simulink library "SEL751_SignalScaling_lib"  (Simulink 8.1)
settings: Solver=ode45  StartTime=0.0  StopTime=10.0  RelTol=1e-3
settings Model: Creator=RE25624  LastModifiedBy=re25624

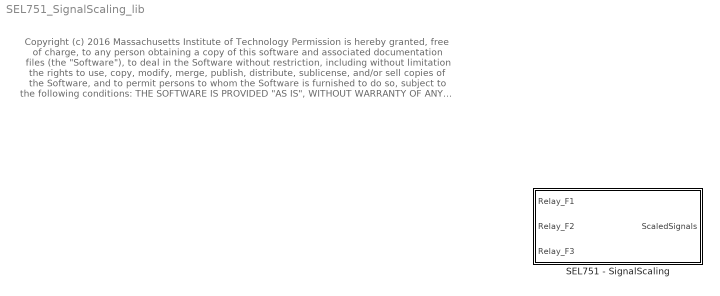
== system SEL751_SignalScaling_lib ==
  note: Copyright (c) 2016 Massachusetts Institute of Technology
      | Permission is hereby granted, free of charge, to any person obtaining a copy of this software and associated documentation files (the "Software"), to deal
      | in the Software without restriction, including without limitation the rights to use, copy, modify, merge, publish, distribute, sublicense, and/or sell copies of the
      | Software, and to permit persons to whom the Software is furnished to do so, subject to the following conditions:
      |
      | THE SOFTWARE IS PROVIDED "AS IS", WITHOUT WARRANTY OF ANY KIND, EXPRESS OR IMPLIED, INCLUDING BUT NOT LIMITED TO THE
      | WARRANTIES OF MERCHANTABILITY, FITNESS FOR A PARTICULAR PURPOSE AND NONINFRINGEMENT. IN NO EVENT SHALL THE AUTHORS
      | OR COPYRIGHT HOLDERS BE LIABLE FOR ANY CLAIM, DAMAGES OR OTHER LIABILITY, WHETHER IN AN ACTION OF CONTRACT, TORT OR
      | OTHERWISE, ARISING FROM, OUT OF OR IN CONNECTION WITH THE SOFTWARE OR THE USE OR OTHER DEALINGS IN THE SOFTWARE
  SEL751 - SignalScaling : Subsystem  mask(SEL751 - SignalScaling){ct_ratio=1/1250, pt_ratio=1/1800}
      mask prompts: ct_ratio "CT Ratio"; pt_ratio "PT Ratio"
      mask help: CT and PT ratios should match the settings in the corresponding SEL751

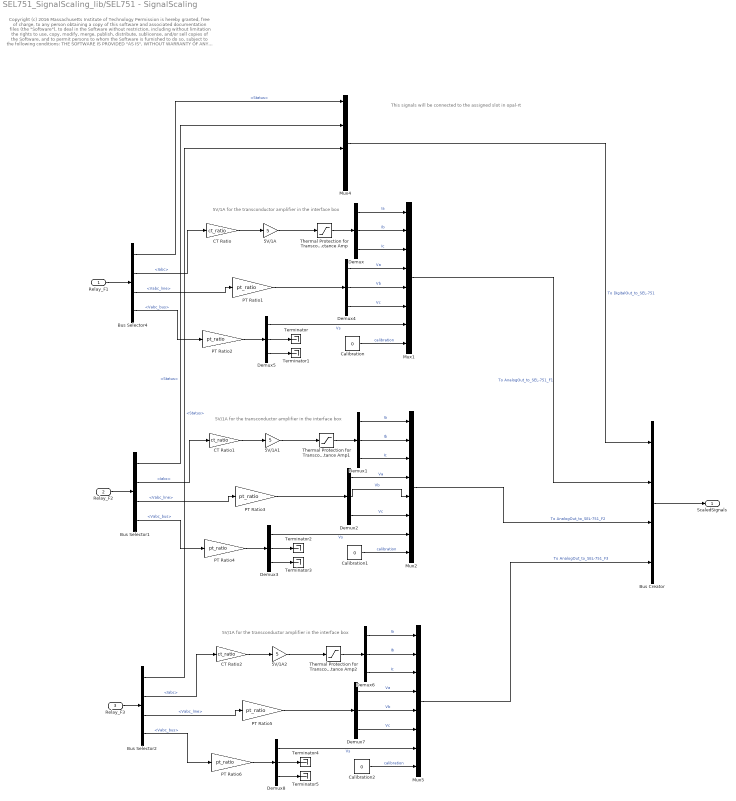
== system SEL751_SignalScaling_lib/SEL751 - SignalScaling ==
  note: Copyright (c) 2016 Massachusetts Institute of Technology
      | Permission is hereby granted, free of charge, to any person obtaining a copy of this software and associated documentation files (the "Software"), to deal
      | in the Software without restriction, including without limitation the rights to use, copy, modify, merge, publish, distribute, sublicense, and/or sell copies of the
      | Software, and to permit persons to whom the Software is furnished to do so, subject to the following conditions:
      |
      | THE SOFTWARE IS PROVIDED "AS IS", WITHOUT WARRANTY OF ANY KIND, EXPRESS OR IMPLIED, INCLUDING BUT NOT LIMITED TO THE
      | WARRANTIES OF MERCHANTABILITY, FITNESS FOR A PARTICULAR PURPOSE AND NONINFRINGEMENT. IN NO EVENT SHALL THE AUTHORS
      | OR COPYRIGHT HOLDERS BE LIABLE FOR ANY CLAIM, DAMAGES OR OTHER LIABILITY, WHETHER IN AN ACTION OF CONTRACT, TORT OR
      | OTHERWISE, ARISING FROM, OUT OF OR IN CONNECTION WITH THE SOFTWARE OR THE USE OR OTHER DEALINGS IN THE SOFTWARE
  note: This signals will be connected to the assigned slot in opal-rt
  note: 5V/1A for the transconductor
      | amplifier in the interface box
  note: 5V/1A for the transconductor
      | amplifier in the interface box
  note: 5V/1A for the transconductor
      | amplifier in the interface box
  Relay_F1 : Inport
  Relay_F2 : Inport  Port=2
  Relay_F3 : Inport  Port=3
  5V/1A : Gain  Gain=5
  5V/1A1 : Gain  Gain=5
  5V/1A2 : Gain  Gain=5
  Bus Creator : BusCreator
  Bus Selector1 : BusSelector  OutputSignals=Status,Iabc,Vabc_line,Vabc_bus
  Bus Selector2 : BusSelector  OutputSignals=Status,Iabc,Vabc_line,Vabc_bus
  Bus Selector4 : BusSelector  OutputSignals=Status,Iabc,Vabc_line,Vabc_bus
  CT Ratio : Gain  Gain=ct_ratio
  CT Ratio1 : Gain  Gain=ct_ratio
  CT Ratio2 : Gain  Gain=ct_ratio
  Calibration : Constant  Value=0
  Calibration1 : Constant  Value=0
  Calibration2 : Constant  Value=0
  Demux{,1..8} (9 alike) : Demux  Outputs=3
  Mux{1..2,4..5} (4 alike) : Mux  Inputs=8
  PT Ratio{1..6} (6 alike) : Gain  Gain=pt_ratio
  Terminator{,1..5} (6 alike) : Terminator
  Thermal Protection for Transconductance Amp : Saturate  UpperLimit=5  LowerLimit=-5
  Thermal Protection for Transconductance Amp1 : Saturate  UpperLimit=5  LowerLimit=-5
  Thermal Protection for Transconductance Amp2 : Saturate  UpperLimit=5  LowerLimit=-5
  ScaledSignals : Outport
  wires:
  5V/1A/1 -> Thermal Protection for Transconductance Amp/1
  Bus Creator/1 -> ScaledSignals/1
  Demux5/3 -> Terminator1/1
  Demux5/2 -> Terminator/1
  Thermal Protection for Transconductance Amp/1 -> Demux/1
  PT Ratio2/1 -> Demux5/1
  PT Ratio1/1 -> Demux4/1
  CT Ratio/1 -> 5V/1A/1
  Relay_F1/1 -> Bus Selector4/1
  Demux/2 -> Mux1/2  "Ib"
  Demux/3 -> Mux1/3  "Ic"
  Demux/1 -> Mux1/1  "Ia"
  Mux1/1 -> Bus Creator/2  "To AnalogOut_to_SEL-751_F1"
  Mux4/1 -> Bus Creator/1  "To DigitalOut_to_SEL-751"
  Bus Selector4/1 -> Mux4/1  "<Status>"
  Calibration/1 -> Mux1/8  "calibration"
  Bus Selector4/3 -> PT Ratio1/1  "<Vabc_line>"
  Demux5/1 -> Mux1/7  "Vs"
  Bus Selector4/4 -> PT Ratio2/1  "<Vabc_bus>"
  Demux4/3 -> Mux1/6  "Vc"
  Demux4/2 -> Mux1/5  "Vb"
  Demux4/1 -> Mux1/4  "Va"
  Bus Selector4/2 -> CT Ratio/1  "<Iabc>"
  5V/1A1/1 -> Thermal Protection for Transconductance Amp1/1
  Demux3/3 -> Terminator3/1
  Demux3/2 -> Terminator2/1
  Thermal Protection for Transconductance Amp1/1 -> Demux1/1
  PT Ratio4/1 -> Demux3/1
  PT Ratio3/1 -> Demux2/1
  CT Ratio1/1 -> 5V/1A1/1
  Demux1/2 -> Mux2/2  "Ib"
  Demux1/3 -> Mux2/3  "Ic"
  Demux1/1 -> Mux2/1  "Ia"
  Mux2/1 -> Bus Creator/3  "To AnalogOut_to_SEL-751_F2"
  Bus Selector1/1 -> Mux4/3  "<Status>"
  Calibration1/1 -> Mux2/8  "calibration"
  Bus Selector1/3 -> PT Ratio3/1  "<Vabc_line>"
  Demux3/1 -> Mux2/7  "Vs"
  Bus Selector1/4 -> PT Ratio4/1  "<Vabc_bus>"
  Demux2/3 -> Mux2/6  "Vc"
  Demux2/2 -> Mux2/5  "Vb"
  Demux2/1 -> Mux2/4  "Va"
  Bus Selector1/2 -> CT Ratio1/1  "<Iabc>"
  5V/1A2/1 -> Thermal Protection for Transconductance Amp2/1
  Demux8/3 -> Terminator5/1
  Demux8/2 -> Terminator4/1
  Thermal Protection for Transconductance Amp2/1 -> Demux6/1
  PT Ratio6/1 -> Demux8/1
  PT Ratio5/1 -> Demux7/1
  CT Ratio2/1 -> 5V/1A2/1
  Demux6/2 -> Mux5/2  "Ib"
  Demux6/3 -> Mux5/3  "Ic"
  Demux6/1 -> Mux5/1  "Ia"
  Mux5/1 -> Bus Creator/4  "To AnalogOut_to_SEL-751_F3"
  Bus Selector2/1 -> Mux4/5  "<Status>"
  Calibration2/1 -> Mux5/8  "calibration"
  Bus Selector2/3 -> PT Ratio5/1  "<Vabc_line>"
  Demux8/1 -> Mux5/7  "Vs"
  Bus Selector2/4 -> PT Ratio6/1  "<Vabc_bus>"
  Demux7/3 -> Mux5/6  "Vc"
  Demux7/2 -> Mux5/5  "Vb"
  Demux7/1 -> Mux5/4  "Va"
  Bus Selector2/2 -> CT Ratio2/1  "<Iabc>"
  Relay_F2/1 -> Bus Selector1/1
  Relay_F3/1 -> Bus Selector2/1
